simulink model "aavs1_8ap"  (R2013a)
settings: Solver=ode45  StartTime=0.0  StopTime=10.0  RelTol=1e-3
undefined symbols (not defined in the file or in its folder): sfp
libraries: xbsIndex_r4 x1437, casper_library_misc x32, xps_library x17
(part 1 of 11)
settings Model: Creator=jack  LastModifiedBy=jack

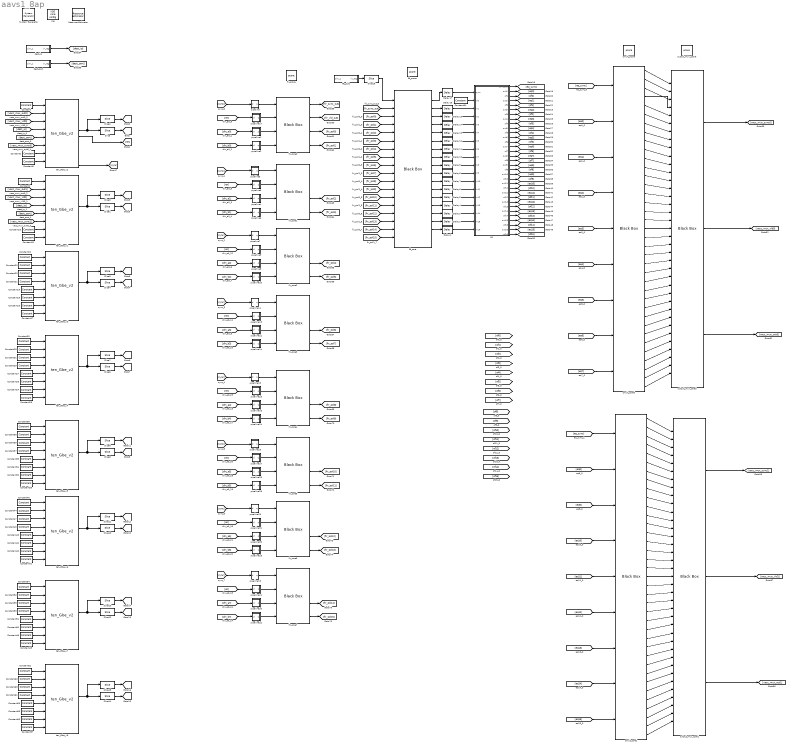
== system aavs1_8ap ==
  " System Generator" : xbsIndex_r4/ System Generator  Tag=genX  xilinxfamily=virtex6  part=xc6vsx475t  speed=-1  package=ff1759  synthesis_tool=XST  clock_wrapper=Clock Enables  directory=./aavs1_8ap/sysgen  proj_type=Project Navigator  Synth_file=XST Defaults  Impl_file=ISE Defaults  testbench=off  simulink_period=1  sysclk_period=5  dcm_input_clock_period=100  incr_netlist=off  trim_vbits=Everywhere in SubSystem  dbl_ovrd=According to Block Masks  core_generation=According to Block Masks  run_coregen=off  deprecated_control=off  eval_field=0  block_type=sysgen
  Constant{,1,18,22..23,26,30..31,34,38..39,42,46..47,50,54..55,58,62..63} (20 alike) : xbsIndex_r4/Constant  const=0  gui_display_data_type=Boolean  arith_type=Boolean  n_bits=16  bin_pt=14  preci_type=Single  exp_width=8  frac_width=24  explicit_period=on  period=1  equ=P=C  opselect=C  inp2=PCIN>>17  opr=+  inp1=P  carry=CIN  dbl_ovrd=off  block_type=constant
  Constant{2..3,10..11,16..17,24..25,32..33,40..41,48..49,56..57,64} (17 alike) : xbsIndex_r4/Constant  const=1  gui_display_data_type=Boolean  arith_type=Boolean  n_bits=16  bin_pt=14  preci_type=Single  exp_width=8  frac_width=24  explicit_period=on  period=1  equ=P=C  opselect=C  inp2=PCIN>>17  opr=+  inp1=P  carry=CIN  dbl_ovrd=off  block_type=constant
  Constant{19,21,27,29,35,37,43,45,51,53,59,61} (12 alike) : xbsIndex_r4/Constant  const=0  gui_display_data_type=Fixed-point  arith_type=Unsigned  n_bits=32  bin_pt=0  preci_type=Single  exp_width=8  frac_width=24  explicit_period=on  period=1  equ=P=C  opselect=C  inp2=PCIN>>17  opr=+  inp1=P  carry=CIN  dbl_ovrd=off  block_type=constant
  Constant{20,28,36,44,52,60} (6 alike) : xbsIndex_r4/Constant  const=0  gui_display_data_type=Fixed-point  arith_type=Unsigned  n_bits=64  bin_pt=0  preci_type=Single  exp_width=8  frac_width=24  explicit_period=on  period=1  equ=P=C  opselect=C  inp2=PCIN>>17  opr=+  inp1=P  carry=CIN  dbl_ovrd=off  block_type=constant
  Delay{1..17} (17 alike) : xbsIndex_r4/Delay  rst=off  infoeditControl=Selection of Reset will increase slice count due to use of real FFs and instead of SRLs  en=off  latency=1  dbl_ovrd=off  reg_retiming=off  block_type=delay
  Resource Estimator : xbsIndex_r4/Resource Estimator  Tag=resEstTag  Slices=0  FFs=0  BRAMs=0  LUTs=0  IOBs=0  EBMs=0  TBUFs=0  xl_use_estimator_area=off  est_options=Estimate  xl_estimator_area=[0 0 0 0 0 0 0]  block_type=resource_estimator
      settings: AttributesFormatString=Resource\nEstimator
  Slice{,1,4,6,8,10,12,14} (8 alike) : xbsIndex_r4/Slice  nbits=32  boolean_output=off  mode=Lower Bit Location + Width  bit1=0  base1=MSB of Input  bit0=0  base0=LSB of Input  dbl_ovrd=off  block_type=slice
  Slice{2..3,5,7,9,11,13,15} (8 alike) : xbsIndex_r4/Slice  nbits=32  boolean_output=off  mode=Lower Bit Location + Width  bit1=0  base1=MSB of Input  bit0=32  base0=LSB of Input  dbl_ovrd=off  block_type=slice
  Slice16 : xbsIndex_r4/Slice  nbits=10  boolean_output=off  mode=Lower Bit Location + Width  bit1=0  base1=MSB of Input  bit0=0  base0=LSB of Input  dbl_ovrd=off  block_type=slice
  cmult_core0 : xbsIndex_r4/Black Box  init_code=cmult_core_config  sim_method=Inactive  verbose=off  block_type=blackbox2
  cmult_core1 : xbsIndex_r4/Black Box  init_code=cmult_core_config  sim_method=Inactive  verbose=off  block_type=blackbox2
  cmult_pcore : xps_library/pcore  Tag=xps:pcore  pcore_path=cmult_core/cmult_core.ngc
  dest_ip : Subsystem  Tag=xps:sw_reg  AncestorBlock=xps_library/software register  mask(swreg){mode=one value, io_dir=From Processor, io_delay=0, sample_period=1, names=reg, bitwidths=32, arith_types=0, bin_pts=0, sim_port=on, show_format=off}
      mask prompts: io_dir "I/O direction"; io_delay "I/O delay"; sample_period "Sample period"; names "Name:"; bitwidths "Bitwidth:"; arith_types "Type (ufix=0, fix=1, bool=2):"; bin_pts "Binary pt:"; sim_port "Provide sim input/output?"; show_format "Print format string?"
      mask init:
      | swreg_init(gcb)
      settings: AttributesFormatString=1input
      mask TypeOptions mode: one value | fields of equal size | fields of arbitrary size
      mask Callback mode: swreg_cb(gcb);
      mask TypeOptions io_dir: To Processor | From Processor
      mask Callback io_dir:
      | mask_enables = get_param(gcb, 'MaskEnables');
      | mask_names = get_param(gcb, 'MaskNames');
      | if strcmp(get_param(gcb, 'io_dir'), 'To Processor'),
      |     mask_enables{ismember(mask_names, 'sample_period')} = 'off';
      | else
      |     mask_enables{ismember(mask_names, 'sample_period')} = 'on';
      | end
      | set_param(gcb, 'MaskEnables', mask_enables);
      mask Callback bitwidths:
      | swreg_maskcheck(gcb);
      | % blk = gcb;
      | % mode = get_param(blk, 'mode');
      | % current_widths = eval(get_param(blk, 'bitwidths'));
      | % if (strcmp(mode, 'one value') || strcmp(mode, 'fields of equal size')) && (length(current_widths) > 1),
      | %     error('Only one width may be specified for this mode.');
      | % elseif strcmp(mode, 'fields of arbitrary size')
      | %     current_names = textscan(strtrim(strrep(strrep(get_param(blk, 'names'), ']', ''), '[', '')), '%s');
      | %     current_names = current_names{1};
      | %     numios = length(current_names);
      | %     if length(current_widths) ~= numios,
      | %         error('%d field names specified, but %d widths?', numios, length(current_widths));
      | %     end
      | % end
      | % total_width = 0;
      | % for ctr = 1 : length(current_widths),
      | %     total_width = total_width + current_widths(ctr);
      | % end
      | % if total_width > 32,
      | %     error('Total width must be 32 or less, set to %d.', total_width);
      | % end
      mask Callback arith_types:
      | [numios, ~, ~, ~, current_types] = swreg_maskcheck(gcb);
      | % blk = gcb;
      | % mode = get_param(blk, 'mode');
      | % current_types = eval(get_param(blk, 'arith_types'));
      | % numios = length(current_types);
      | % if (strcmp(mode, 'one value') || strcmp(mode, 'fields of equal size')) && (length(current_types) > 1),
      | %     error('Only one type may be specified for this mode.');
      | % elseif strcmp(mode, 'fields of arbitrary size')
      | %     current_names = textscan(strtrim(strrep(strrep(get_param(blk, 'names'), ']', ''), '[', '')), '%s');
      | %     current_names = current_names{1};
      | %     numios = length(current_names);
      | %     if length(current_types) ~= numios,
      | %         error('%d field names specified, but %d types?', numios, length(current_types));
      | %     end
      | % end
      | problem = 0;
      | for ctr = 1 : numios,
      |     t = current_types(ctr);
      |     if (t < 0) || (t > 2),
      |         problem = t;
      |         ctr = numios + 1;
      |     end
      | end
      | if problem ~= 0,
      |     error('Type cannot be %i, must be 0, 1 or 2.', problem);
      | end
      mask Callback bin_pts:
      | swreg_maskcheck(gcb);
      | % blk = gcb;
      | % mode = get_param(blk, 'mode');
      | % current_bins = eval(get_param(blk, 'bin_pts'));
      | % if (strcmp(mode, 'one value') || strcmp(mode, 'fields of equal size')) && (length(current_bins) > 1),
      | %     error('Only one binary pt may be specified for this mode.');
      | % elseif strcmp(mode, 'fields of arbitrary size')
      | %     current_names = textscan(strtrim(strrep(strrep(get_param(blk, 'names'), ']', ''), '[', '')), '%s');
      | %     current_names = current_names{1};
      | %     numios = length(current_names);
      | %     if length(current_bins) ~= numios,
      | %         error('%d field names specified, but %d binary pts?', numios, length(current_bins));
      | %     end
      | % end
  dest_port : Subsystem  Tag=xps:sw_reg  AncestorBlock=xps_library/software register  mask(swreg){mode=one value, io_dir=From Processor, io_delay=0, sample_period=1, names=reg, bitwidths=32, arith_types=0, bin_pts=0, sim_port=on, show_format=off}
      mask prompts: io_dir "I/O direction"; io_delay "I/O delay"; sample_period "Sample period"; names "Name:"; bitwidths "Bitwidth:"; arith_types "Type (ufix=0, fix=1, bool=2):"; bin_pts "Binary pt:"; sim_port "Provide sim input/output?"; show_format "Print format string?"
      mask init:
      | swreg_init(gcb)
      settings: AttributesFormatString=1input
      mask TypeOptions mode: one value | fields of equal size | fields of arbitrary size
      mask Callback mode: swreg_cb(gcb);
      mask TypeOptions io_dir: To Processor | From Processor
      mask Callback io_dir:
      | mask_enables = get_param(gcb, 'MaskEnables');
      | mask_names = get_param(gcb, 'MaskNames');
      | if strcmp(get_param(gcb, 'io_dir'), 'To Processor'),
      |     mask_enables{ismember(mask_names, 'sample_period')} = 'off';
      | else
      |     mask_enables{ismember(mask_names, 'sample_period')} = 'on';
      | end
      | set_param(gcb, 'MaskEnables', mask_enables);
      mask Callback bitwidths:
      | swreg_maskcheck(gcb);
      | % blk = gcb;
      | % mode = get_param(blk, 'mode');
      | % current_widths = eval(get_param(blk, 'bitwidths'));
      | % if (strcmp(mode, 'one value') || strcmp(mode, 'fields of equal size')) && (length(current_widths) > 1),
      | %     error('Only one width may be specified for this mode.');
      | % elseif strcmp(mode, 'fields of arbitrary size')
      | %     current_names = textscan(strtrim(strrep(strrep(get_param(blk, 'names'), ']', ''), '[', '')), '%s');
      | %     current_names = current_names{1};
      | %     numios = length(current_names);
      | %     if length(current_widths) ~= numios,
      | %         error('%d field names specified, but %d widths?', numios, length(current_widths));
      | %     end
      | % end
      | % total_width = 0;
      | % for ctr = 1 : length(current_widths),
      | %     total_width = total_width + current_widths(ctr);
      | % end
      | % if total_width > 32,
      | %     error('Total width must be 32 or less, set to %d.', total_width);
      | % end
      mask Callback arith_types:
      | [numios, ~, ~, ~, current_types] = swreg_maskcheck(gcb);
      | % blk = gcb;
      | % mode = get_param(blk, 'mode');
      | % current_types = eval(get_param(blk, 'arith_types'));
      | % numios = length(current_types);
      | % if (strcmp(mode, 'one value') || strcmp(mode, 'fields of equal size')) && (length(current_types) > 1),
      | %     error('Only one type may be specified for this mode.');
      | % elseif strcmp(mode, 'fields of arbitrary size')
      | %     current_names = textscan(strtrim(strrep(strrep(get_param(blk, 'names'), ']', ''), '[', '')), '%s');
      | %     current_names = current_names{1};
      | %     numios = length(current_names);
      | %     if length(current_types) ~= numios,
      | %         error('%d field names specified, but %d types?', numios, length(current_types));
      | %     end
      | % end
      | problem = 0;
      | for ctr = 1 : numios,
      |     t = current_types(ctr);
      |     if (t < 0) || (t > 2),
      |         problem = t;
      |         ctr = numios + 1;
      |     end
      | end
      | if problem ~= 0,
      |     error('Type cannot be %i, must be 0, 1 or 2.', problem);
      | end
      mask Callback bin_pts:
      | swreg_maskcheck(gcb);
      | % blk = gcb;
      | % mode = get_param(blk, 'mode');
      | % current_bins = eval(get_param(blk, 'bin_pts'));
      | % if (strcmp(mode, 'one value') || strcmp(mode, 'fields of equal size')) && (length(current_bins) > 1),
      | %     error('Only one binary pt may be specified for this mode.');
      | % elseif strcmp(mode, 'fields of arbitrary size')
      | %     current_names = textscan(strtrim(strrep(strrep(get_param(blk, 'names'), ']', ''), '[', '')), '%s');
      | %     current_names = current_names{1};
      | %     numios = length(current_names);
      | %     if length(current_bins) ~= numios,
      | %         error('%d field names specified, but %d binary pts?', numios, length(current_bins));
      | %     end
      | % end
  eq : Subsystem
  fft_core : xbsIndex_r4/Black Box  init_code=fft_core_config  sim_method=Inactive  verbose=off  block_type=blackbox2
  fft_pcore : xps_library/pcore  Tag=xps:pcore  pcore_path=fft_core/fft_core.ngc
  fft_shift : Subsystem  Tag=xps:sw_reg  AncestorBlock=xps_library/software register  mask(swreg){mode=one value, io_dir=From Processor, io_delay=0, sample_period=1, names=reg, bitwidths=32, arith_types=0, bin_pts=0, sim_port=on, show_format=off}
      mask prompts: io_dir "I/O direction"; io_delay "I/O delay"; sample_period "Sample period"; names "Name:"; bitwidths "Bitwidth:"; arith_types "Type (ufix=0, fix=1, bool=2):"; bin_pts "Binary pt:"; sim_port "Provide sim input/output?"; show_format "Print format string?"
      mask init:
      | swreg_init(gcb)
      settings: AttributesFormatString=1input
      mask TypeOptions mode: one value | fields of equal size | fields of arbitrary size
      mask Callback mode: swreg_cb(gcb);
      mask TypeOptions io_dir: To Processor | From Processor
      mask Callback io_dir:
      | mask_enables = get_param(gcb, 'MaskEnables');
      | mask_names = get_param(gcb, 'MaskNames');
      | if strcmp(get_param(gcb, 'io_dir'), 'To Processor'),
      |     mask_enables{ismember(mask_names, 'sample_period')} = 'off';
      | else
      |     mask_enables{ismember(mask_names, 'sample_period')} = 'on';
      | end
      | set_param(gcb, 'MaskEnables', mask_enables);
      mask Callback bitwidths:
      | swreg_maskcheck(gcb);
      | % blk = gcb;
      | % mode = get_param(blk, 'mode');
      | % current_widths = eval(get_param(blk, 'bitwidths'));
      | % if (strcmp(mode, 'one value') || strcmp(mode, 'fields of equal size')) && (length(current_widths) > 1),
      | %     error('Only one width may be specified for this mode.');
      | % elseif strcmp(mode, 'fields of arbitrary size')
      | %     current_names = textscan(strtrim(strrep(strrep(get_param(blk, 'names'), ']', ''), '[', '')), '%s');
      | %     current_names = current_names{1};
      | %     numios = length(current_names);
      | %     if length(current_widths) ~= numios,
      | %         error('%d field names specified, but %d widths?', numios, length(current_widths));
      | %     end
      | % end
      | % total_width = 0;
      | % for ctr = 1 : length(current_widths),
      | %     total_width = total_width + current_widths(ctr);
      | % end
      | % if total_width > 32,
      | %     error('Total width must be 32 or less, set to %d.', total_width);
      | % end
      mask Callback arith_types:
      | [numios, ~, ~, ~, current_types] = swreg_maskcheck(gcb);
      | % blk = gcb;
      | % mode = get_param(blk, 'mode');
      | % current_types = eval(get_param(blk, 'arith_types'));
      | % numios = length(current_types);
      | % if (strcmp(mode, 'one value') || strcmp(mode, 'fields of equal size')) && (length(current_types) > 1),
      | %     error('Only one type may be specified for this mode.');
      | % elseif strcmp(mode, 'fields of arbitrary size')
      | %     current_names = textscan(strtrim(strrep(strrep(get_param(blk, 'names'), ']', ''), '[', '')), '%s');
      | %     current_names = current_names{1};
      | %     numios = length(current_names);
      | %     if length(current_types) ~= numios,
      | %         error('%d field names specified, but %d types?', numios, length(current_types));
      | %     end
      | % end
      | problem = 0;
      | for ctr = 1 : numios,
      |     t = current_types(ctr);
      |     if (t < 0) || (t > 2),
      |         problem = t;
      |         ctr = numios + 1;
      |     end
      | end
      | if problem ~= 0,
      |     error('Type cannot be %i, must be 0, 1 or 2.', problem);
      | end
      mask Callback bin_pts:
      | swreg_maskcheck(gcb);
      | % blk = gcb;
      | % mode = get_param(blk, 'mode');
      | % current_bins = eval(get_param(blk, 'bin_pts'));
      | % if (strcmp(mode, 'one value') || strcmp(mode, 'fields of equal size')) && (length(current_bins) > 1),
      | %     error('Only one binary pt may be specified for this mode.');
      | % elseif strcmp(mode, 'fields of arbitrary size')
      | %     current_names = textscan(strtrim(strrep(strrep(get_param(blk, 'names'), ']', ''), '[', '')), '%s');
      | %     current_names = current_names{1};
      | %     numios = length(current_names);
      | %     if length(current_bins) ~= numios,
      | %         error('%d field names specified, but %d binary pts?', numios, length(current_bins));
      | %     end
      | % end
  fir_core{0..7} (8 alike) : xbsIndex_r4/Black Box  init_code=fir_core_config  sim_method=Inactive  verbose=off  block_type=blackbox2
  fir_pcore : xps_library/pcore  Tag=xps:pcore  pcore_path=fir_core/fir_core.ngc
  output_mux_core0 : xbsIndex_r4/Black Box  init_code=output_mux_core_config  sim_method=Inactive  verbose=off  block_type=blackbox2
  output_mux_core1 : xbsIndex_r4/Black Box  init_code=output_mux_core_config  sim_method=Inactive  verbose=off  block_type=blackbox2
  output_mux_pcore : xps_library/pcore  Tag=xps:pcore  pcore_path=output_mux_core/output_mux_core.ngc
  pipeline : Subsystem  AncestorBlock=casper_library_delays/pipeline  mask(pipeline){latency=1}
      mask help:
      | An explicitly laid-out delay line to avoid mapping to SRL16s
      | for use in pipelining to help achieve timing closure.
      mask init:
      | pipeline_init(gcb,'latency',latency);
      settings: AttributesFormatString=Latency = %<latency>
      mask Display:
      | port_label('input', 1, 'd');
      | port_label('output', 1, 'q');
      | disp(['Z^-', num2str(latency)]);
  pipeline1 : Subsystem  AncestorBlock=casper_library_delays/pipeline  mask(pipeline){latency=1}
      mask help:
      | An explicitly laid-out delay line to avoid mapping to SRL16s
      | for use in pipelining to help achieve timing closure.
      mask init:
      | pipeline_init(gcb,'latency',latency);
      settings: AttributesFormatString=Latency = %<latency>
      mask Display:
      | port_label('input', 1, 'd');
      | port_label('output', 1, 'q');
      | disp(['Z^-', num2str(latency)]);
  pipeline10 : Subsystem  AncestorBlock=casper_library_delays/pipeline  mask(pipeline){latency=1}
      mask help:
      | An explicitly laid-out delay line to avoid mapping to SRL16s
      | for use in pipelining to help achieve timing closure.
      mask init:
      | pipeline_init(gcb,'latency',latency);
      settings: AttributesFormatString=Latency = %<latency>
      mask Display:
      | port_label('input', 1, 'd');
      | port_label('output', 1, 'q');
      | disp(['Z^-', num2str(latency)]);
  pipeline11 : Subsystem  AncestorBlock=casper_library_delays/pipeline  mask(pipeline){latency=1}
      mask help:
      | An explicitly laid-out delay line to avoid mapping to SRL16s
      | for use in pipelining to help achieve timing closure.
      mask init:
      | pipeline_init(gcb,'latency',latency);
      settings: AttributesFormatString=Latency = %<latency>
      mask Display:
      | port_label('input', 1, 'd');
      | port_label('output', 1, 'q');
      | disp(['Z^-', num2str(latency)]);
  pipeline12 : Subsystem  AncestorBlock=casper_library_delays/pipeline  mask(pipeline){latency=1}
      mask help:
      | An explicitly laid-out delay line to avoid mapping to SRL16s
      | for use in pipelining to help achieve timing closure.
      mask init:
      | pipeline_init(gcb,'latency',latency);
      settings: AttributesFormatString=Latency = %<latency>
      mask Display:
      | port_label('input', 1, 'd');
      | port_label('output', 1, 'q');
      | disp(['Z^-', num2str(latency)]);
  pipeline13 : Subsystem  AncestorBlock=casper_library_delays/pipeline  mask(pipeline){latency=1}
      mask help:
      | An explicitly laid-out delay line to avoid mapping to SRL16s
      | for use in pipelining to help achieve timing closure.
      mask init:
      | pipeline_init(gcb,'latency',latency);
      settings: AttributesFormatString=Latency = %<latency>
      mask Display:
      | port_label('input', 1, 'd');
      | port_label('output', 1, 'q');
      | disp(['Z^-', num2str(latency)]);
  pipeline14 : Subsystem  AncestorBlock=casper_library_delays/pipeline  mask(pipeline){latency=1}
      mask help:
      | An explicitly laid-out delay line to avoid mapping to SRL16s
      | for use in pipelining to help achieve timing closure.
      mask init:
      | pipeline_init(gcb,'latency',latency);
      settings: AttributesFormatString=Latency = %<latency>
      mask Display:
      | port_label('input', 1, 'd');
      | port_label('output', 1, 'q');
      | disp(['Z^-', num2str(latency)]);
  pipeline15 : Subsystem  AncestorBlock=casper_library_delays/pipeline  mask(pipeline){latency=1}
      mask help:
      | An explicitly laid-out delay line to avoid mapping to SRL16s
      | for use in pipelining to help achieve timing closure.
      mask init:
      | pipeline_init(gcb,'latency',latency);
      settings: AttributesFormatString=Latency = %<latency>
      mask Display:
      | port_label('input', 1, 'd');
      | port_label('output', 1, 'q');
      | disp(['Z^-', num2str(latency)]);
  pipeline16 : Subsystem  AncestorBlock=casper_library_delays/pipeline  mask(pipeline){latency=1}
      mask help:
      | An explicitly laid-out delay line to avoid mapping to SRL16s
      | for use in pipelining to help achieve timing closure.
      mask init:
      | pipeline_init(gcb,'latency',latency);
      settings: AttributesFormatString=Latency = %<latency>
      mask Display:
      | port_label('input', 1, 'd');
      | port_label('output', 1, 'q');
      | disp(['Z^-', num2str(latency)]);
  pipeline17 : Subsystem  AncestorBlock=casper_library_delays/pipeline  mask(pipeline){latency=1}
      mask help:
      | An explicitly laid-out delay line to avoid mapping to SRL16s
      | for use in pipelining to help achieve timing closure.
      mask init:
      | pipeline_init(gcb,'latency',latency);
      settings: AttributesFormatString=Latency = %<latency>
      mask Display:
      | port_label('input', 1, 'd');
      | port_label('output', 1, 'q');
      | disp(['Z^-', num2str(latency)]);
  pipeline18 : Subsystem  AncestorBlock=casper_library_delays/pipeline  mask(pipeline){latency=1}
      mask help:
      | An explicitly laid-out delay line to avoid mapping to SRL16s
      | for use in pipelining to help achieve timing closure.
      mask init:
      | pipeline_init(gcb,'latency',latency);
      settings: AttributesFormatString=Latency = %<latency>
      mask Display:
      | port_label('input', 1, 'd');
      | port_label('output', 1, 'q');
      | disp(['Z^-', num2str(latency)]);
  pipeline19 : Subsystem  AncestorBlock=casper_library_delays/pipeline  mask(pipeline){latency=1}
      mask help:
      | An explicitly laid-out delay line to avoid mapping to SRL16s
      | for use in pipelining to help achieve timing closure.
      mask init:
      | pipeline_init(gcb,'latency',latency);
      settings: AttributesFormatString=Latency = %<latency>
      mask Display:
      | port_label('input', 1, 'd');
      | port_label('output', 1, 'q');
      | disp(['Z^-', num2str(latency)]);
  pipeline2 : Subsystem  AncestorBlock=casper_library_delays/pipeline  mask(pipeline){latency=1}
      mask help:
      | An explicitly laid-out delay line to avoid mapping to SRL16s
      | for use in pipelining to help achieve timing closure.
      mask init:
      | pipeline_init(gcb,'latency',latency);
      settings: AttributesFormatString=Latency = %<latency>
      mask Display:
      | port_label('input', 1, 'd');
      | port_label('output', 1, 'q');
      | disp(['Z^-', num2str(latency)]);
  pipeline20 : Subsystem  AncestorBlock=casper_library_delays/pipeline  mask(pipeline){latency=1}
      mask help:
      | An explicitly laid-out delay line to avoid mapping to SRL16s
      | for use in pipelining to help achieve timing closure.
      mask init:
      | pipeline_init(gcb,'latency',latency);
      settings: AttributesFormatString=Latency = %<latency>
      mask Display:
      | port_label('input', 1, 'd');
      | port_label('output', 1, 'q');
      | disp(['Z^-', num2str(latency)]);
  pipeline21 : Subsystem  AncestorBlock=casper_library_delays/pipeline  mask(pipeline){latency=1}
      mask help:
      | An explicitly laid-out delay line to avoid mapping to SRL16s
      | for use in pipelining to help achieve timing closure.
      mask init:
      | pipeline_init(gcb,'latency',latency);
      settings: AttributesFormatString=Latency = %<latency>
      mask Display:
      | port_label('input', 1, 'd');
      | port_label('output', 1, 'q');
      | disp(['Z^-', num2str(latency)]);
  pipeline22 : Subsystem  AncestorBlock=casper_library_delays/pipeline  mask(pipeline){latency=1}
      mask help:
      | An explicitly laid-out delay line to avoid mapping to SRL16s
      | for use in pipelining to help achieve timing closure.
      mask init:
      | pipeline_init(gcb,'latency',latency);
      settings: AttributesFormatString=Latency = %<latency>
      mask Display:
      | port_label('input', 1, 'd');
      | port_label('output', 1, 'q');
      | disp(['Z^-', num2str(latency)]);
  pipeline23 : Subsystem  AncestorBlock=casper_library_delays/pipeline  mask(pipeline){latency=1}
      mask help:
      | An explicitly laid-out delay line to avoid mapping to SRL16s
      | for use in pipelining to help achieve timing closure.
      mask init:
      | pipeline_init(gcb,'latency',latency);
      settings: AttributesFormatString=Latency = %<latency>
      mask Display:
      | port_label('input', 1, 'd');
      | port_label('output', 1, 'q');
      | disp(['Z^-', num2str(latency)]);
  pipeline24 : Subsystem  AncestorBlock=casper_library_delays/pipeline  mask(pipeline){latency=1}
      mask help:
      | An explicitly laid-out delay line to avoid mapping to SRL16s
      | for use in pipelining to help achieve timing closure.
      mask init:
      | pipeline_init(gcb,'latency',latency);
      settings: AttributesFormatString=Latency = %<latency>
      mask Display:
      | port_label('input', 1, 'd');
      | port_label('output', 1, 'q');
      | disp(['Z^-', num2str(latency)]);
  pipeline25 : Subsystem  AncestorBlock=casper_library_delays/pipeline  mask(pipeline){latency=1}
      mask help:
      | An explicitly laid-out delay line to avoid mapping to SRL16s
      | for use in pipelining to help achieve timing closure.
      mask init:
      | pipeline_init(gcb,'latency',latency);
      settings: AttributesFormatString=Latency = %<latency>
      mask Display:
      | port_label('input', 1, 'd');
      | port_label('output', 1, 'q');
      | disp(['Z^-', num2str(latency)]);
  pipeline26 : Subsystem  AncestorBlock=casper_library_delays/pipeline  mask(pipeline){latency=1}
      mask help:
      | An explicitly laid-out delay line to avoid mapping to SRL16s
      | for use in pipelining to help achieve timing closure.
      mask init:
      | pipeline_init(gcb,'latency',latency);
      settings: AttributesFormatString=Latency = %<latency>
      mask Display:
      | port_label('input', 1, 'd');
      | port_label('output', 1, 'q');
      | disp(['Z^-', num2str(latency)]);
  pipeline27 : Subsystem  AncestorBlock=casper_library_delays/pipeline  mask(pipeline){latency=1}
      mask help:
      | An explicitly laid-out delay line to avoid mapping to SRL16s
      | for use in pipelining to help achieve timing closure.
      mask init:
      | pipeline_init(gcb,'latency',latency);
      settings: AttributesFormatString=Latency = %<latency>
      mask Display:
      | port_label('input', 1, 'd');
      | port_label('output', 1, 'q');
      | disp(['Z^-', num2str(latency)]);
  pipeline28 : Subsystem  AncestorBlock=casper_library_delays/pipeline  mask(pipeline){latency=1}
      mask help:
      | An explicitly laid-out delay line to avoid mapping to SRL16s
      | for use in pipelining to help achieve timing closure.
      mask init:
      | pipeline_init(gcb,'latency',latency);
      settings: AttributesFormatString=Latency = %<latency>
      mask Display:
      | port_label('input', 1, 'd');
      | port_label('output', 1, 'q');
      | disp(['Z^-', num2str(latency)]);
  pipeline29 : Subsystem  AncestorBlock=casper_library_delays/pipeline  mask(pipeline){latency=1}
      mask help:
      | An explicitly laid-out delay line to avoid mapping to SRL16s
      | for use in pipelining to help achieve timing closure.
      mask init:
      | pipeline_init(gcb,'latency',latency);
      settings: AttributesFormatString=Latency = %<latency>
      mask Display:
      | port_label('input', 1, 'd');
      | port_label('output', 1, 'q');
      | disp(['Z^-', num2str(latency)]);
  pipeline3 : Subsystem  AncestorBlock=casper_library_delays/pipeline  mask(pipeline){latency=1}
      mask help:
      | An explicitly laid-out delay line to avoid mapping to SRL16s
      | for use in pipelining to help achieve timing closure.
      mask init:
      | pipeline_init(gcb,'latency',latency);
      settings: AttributesFormatString=Latency = %<latency>
      mask Display:
      | port_label('input', 1, 'd');
      | port_label('output', 1, 'q');
      | disp(['Z^-', num2str(latency)]);
  pipeline30 : Subsystem  AncestorBlock=casper_library_delays/pipeline  mask(pipeline){latency=1}
      mask help:
      | An explicitly laid-out delay line to avoid mapping to SRL16s
      | for use in pipelining to help achieve timing closure.
      mask init:
      | pipeline_init(gcb,'latency',latency);
      settings: AttributesFormatString=Latency = %<latency>
      mask Display:
      | port_label('input', 1, 'd');
      | port_label('output', 1, 'q');
      | disp(['Z^-', num2str(latency)]);
  pipeline31 : Subsystem  AncestorBlock=casper_library_delays/pipeline  mask(pipeline){latency=1}
      mask help:
      | An explicitly laid-out delay line to avoid mapping to SRL16s
      | for use in pipelining to help achieve timing closure.
      mask init:
      | pipeline_init(gcb,'latency',latency);
      settings: AttributesFormatString=Latency = %<latency>
      mask Display:
      | port_label('input', 1, 'd');
      | port_label('output', 1, 'q');
      | disp(['Z^-', num2str(latency)]);
  pipeline4 : Subsystem  AncestorBlock=casper_library_delays/pipeline  mask(pipeline){latency=1}
      mask help:
      | An explicitly laid-out delay line to avoid mapping to SRL16s
      | for use in pipelining to help achieve timing closure.
      mask init:
      | pipeline_init(gcb,'latency',latency);
      settings: AttributesFormatString=Latency = %<latency>
      mask Display:
      | port_label('input', 1, 'd');
      | port_label('output', 1, 'q');
      | disp(['Z^-', num2str(latency)]);
  pipeline5 : Subsystem  AncestorBlock=casper_library_delays/pipeline  mask(pipeline){latency=1}
      mask help:
      | An explicitly laid-out delay line to avoid mapping to SRL16s
      | for use in pipelining to help achieve timing closure.
      mask init:
      | pipeline_init(gcb,'latency',latency);
      settings: AttributesFormatString=Latency = %<latency>
      mask Display:
      | port_label('input', 1, 'd');
      | port_label('output', 1, 'q');
      | disp(['Z^-', num2str(latency)]);
  pipeline6 : Subsystem  AncestorBlock=casper_library_delays/pipeline  mask(pipeline){latency=1}
      mask help:
      | An explicitly laid-out delay line to avoid mapping to SRL16s
      | for use in pipelining to help achieve timing closure.
      mask init:
      | pipeline_init(gcb,'latency',latency);
      settings: AttributesFormatString=Latency = %<latency>
      mask Display:
      | port_label('input', 1, 'd');
      | port_label('output', 1, 'q');
      | disp(['Z^-', num2str(latency)]);
  pipeline7 : Subsystem  AncestorBlock=casper_library_delays/pipeline  mask(pipeline){latency=1}
      mask help:
      | An explicitly laid-out delay line to avoid mapping to SRL16s
      | for use in pipelining to help achieve timing closure.
      mask init:
      | pipeline_init(gcb,'latency',latency);
      settings: AttributesFormatString=Latency = %<latency>
      mask Display:
      | port_label('input', 1, 'd');
      | port_label('output', 1, 'q');
      | disp(['Z^-', num2str(latency)]);
  pipeline8 : Subsystem  AncestorBlock=casper_library_delays/pipeline  mask(pipeline){latency=1}
      mask help:
      | An explicitly laid-out delay line to avoid mapping to SRL16s
      | for use in pipelining to help achieve timing closure.
      mask init:
      | pipeline_init(gcb,'latency',latency);
      settings: AttributesFormatString=Latency = %<latency>
      mask Display:
      | port_label('input', 1, 'd');
      | port_label('output', 1, 'q');
      | disp(['Z^-', num2str(latency)]);
  pipeline9 : Subsystem  AncestorBlock=casper_library_delays/pipeline  mask(pipeline){latency=1}
      mask help:
      | An explicitly laid-out delay line to avoid mapping to SRL16s
      | for use in pipelining to help achieve timing closure.
      mask init:
      | pipeline_init(gcb,'latency',latency);
      settings: AttributesFormatString=Latency = %<latency>
      mask Display:
      | port_label('input', 1, 'd');
      | port_label('output', 1, 'q');
      | disp(['Z^-', num2str(latency)]);
  ten_Gbe_v1 : xps_library/ten_Gbe_v2  Tag=xps:tengbe_v2  flavour=sfp+  slot=0  port_r1=0  port_r2_cx4=0  port_r2_sfpp=1  rx_dist_ram=on  large_frames=off  show_param=off  pre_emph_r2=1.07  pre_emph=3  post_emph_r2=0.18  rxeqmix_r2=7  swing_r2=940  swing=800  fab_en=on  fab_mac=hex2dec('123456780000')  fab_ip=192*(2^24) + 168*(2^16) + 5*(2^8) + 20*(2^0)  fab_udp=10000  fab_gate=1  cpu_rx_en=on  cpu_tx_en=on  ttl=hex2dec('FF')  promisc_mode=off  txctr=off  txerrctr=off  txerrctr_len=100  txofctr=off  txfullctr=off  txvldctr=off  txsnaplen=0 - no snap  rxctr=off  rxerrctr=off  rxerrctr_len=100  rxofctr=off  rxbadctr=off  rxvldctr=off  rxeofctr=off  rxsnaplen=0 - no snap
  ten_Gbe_v2 : xps_library/ten_Gbe_v2  Tag=xps:tengbe_v2  flavour=sfp+  slot=0  port_r1=0  port_r2_cx4=0  port_r2_sfpp=0  rx_dist_ram=on  large_frames=off  show_param=off  pre_emph_r2=1.07  pre_emph=3  post_emph_r2=0.18  rxeqmix_r2=7  swing_r2=940  swing=800  fab_en=on  fab_mac=hex2dec('123456780000')  fab_ip=192*(2^24) + 168*(2^16) + 5*(2^8) + 20*(2^0)  fab_udp=10000  fab_gate=1  cpu_rx_en=on  cpu_tx_en=on  ttl=hex2dec('FF')  promisc_mode=off  txctr=off  txerrctr=off  txerrctr_len=100  txofctr=off  txfullctr=off  txvldctr=off  txsnaplen=0 - no snap  rxctr=off  rxerrctr=off  rxerrctr_len=100  rxofctr=off  rxbadctr=off  rxvldctr=off  rxeofctr=off  rxsnaplen=0 - no snap
  ten_Gbe_v3 : xps_library/ten_Gbe_v2  Tag=xps:tengbe_v2  flavour=sfp+  slot=0  port_r1=0  port_r2_cx4=0  port_r2_sfpp=2  rx_dist_ram=on  large_frames=off  show_param=off  pre_emph_r2=1.07  pre_emph=3  post_emph_r2=0.18  rxeqmix_r2=7  swing_r2=940  swing=800  fab_en=on  fab_mac=hex2dec('123456780000')  fab_ip=192*(2^24) + 168*(2^16) + 5*(2^8) + 20*(2^0)  fab_udp=10000  fab_gate=1  cpu_rx_en=on  cpu_tx_en=on  ttl=hex2dec('FF')  promisc_mode=off  txctr=off  txerrctr=off  txerrctr_len=100  txofctr=off  txfullctr=off  txvldctr=off  txsnaplen=0 - no snap  rxctr=off  rxerrctr=off  rxerrctr_len=100  rxofctr=off  rxbadctr=off  rxvldctr=off  rxeofctr=off  rxsnaplen=0 - no snap
  ten_Gbe_v4 : xps_library/ten_Gbe_v2  Tag=xps:tengbe_v2  flavour=sfp+  slot=0  port_r1=0  port_r2_cx4=0  port_r2_sfpp=3  rx_dist_ram=on  large_frames=off  show_param=off  pre_emph_r2=1.07  pre_emph=3  post_emph_r2=0.18  rxeqmix_r2=7  swing_r2=940  swing=800  fab_en=on  fab_mac=hex2dec('123456780000')  fab_ip=192*(2^24) + 168*(2^16) + 5*(2^8) + 20*(2^0)  fab_udp=10000  fab_gate=1  cpu_rx_en=on  cpu_tx_en=on  ttl=hex2dec('FF')  promisc_mode=off  txctr=off  txerrctr=off  txerrctr_len=100  txofctr=off  txfullctr=off  txvldctr=off  txsnaplen=0 - no snap  rxctr=off  rxerrctr=off  rxerrctr_len=100  rxofctr=off  rxbadctr=off  rxvldctr=off  rxeofctr=off  rxsnaplen=0 - no snap
  ten_Gbe_v5 : xps_library/ten_Gbe_v2  Tag=xps:tengbe_v2  flavour=sfp+  slot=1  port_r1=0  port_r2_cx4=0  port_r2_sfpp=0  rx_dist_ram=on  large_frames=off  show_param=off  pre_emph_r2=1.07  pre_emph=3  post_emph_r2=0.18  rxeqmix_r2=7  swing_r2=940  swing=800  fab_en=on  fab_mac=hex2dec('123456780000')  fab_ip=192*(2^24) + 168*(2^16) + 5*(2^8) + 20*(2^0)  fab_udp=10000  fab_gate=1  cpu_rx_en=on  cpu_tx_en=on  ttl=hex2dec('FF')  promisc_mode=off  txctr=off  txerrctr=off  txerrctr_len=100  txofctr=off  txfullctr=off  txvldctr=off  txsnaplen=0 - no snap  rxctr=off  rxerrctr=off  rxerrctr_len=100  rxofctr=off  rxbadctr=off  rxvldctr=off  rxeofctr=off  rxsnaplen=0 - no snap
  ten_Gbe_v6 : xps_library/ten_Gbe_v2  Tag=xps:tengbe_v2  flavour=sfp+  slot=1  port_r1=0  port_r2_cx4=0  port_r2_sfpp=1  rx_dist_ram=on  large_frames=off  show_param=off  pre_emph_r2=1.07  pre_emph=3  post_emph_r2=0.18  rxeqmix_r2=7  swing_r2=940  swing=800  fab_en=on  fab_mac=hex2dec('123456780000')  fab_ip=192*(2^24) + 168*(2^16) + 5*(2^8) + 20*(2^0)  fab_udp=10000  fab_gate=1  cpu_rx_en=on  cpu_tx_en=on  ttl=hex2dec('FF')  promisc_mode=off  txctr=off  txerrctr=off  txerrctr_len=100  txofctr=off  txfullctr=off  txvldctr=off  txsnaplen=0 - no snap  rxctr=off  rxerrctr=off  rxerrctr_len=100  rxofctr=off  rxbadctr=off  rxvldctr=off  rxeofctr=off  rxsnaplen=0 - no snap
  ten_Gbe_v7 : xps_library/ten_Gbe_v2  Tag=xps:tengbe_v2  flavour=sfp+  slot=1  port_r1=0  port_r2_cx4=0  port_r2_sfpp=2  rx_dist_ram=on  large_frames=off  show_param=off  pre_emph_r2=1.07  pre_emph=3  post_emph_r2=0.18  rxeqmix_r2=7  swing_r2=940  swing=800  fab_en=on  fab_mac=hex2dec('123456780000')  fab_ip=192*(2^24) + 168*(2^16) + 5*(2^8) + 20*(2^0)  fab_udp=10000  fab_gate=1  cpu_rx_en=on  cpu_tx_en=on  ttl=hex2dec('FF')  promisc_mode=off  txctr=off  txerrctr=off  txerrctr_len=100  txofctr=off  txfullctr=off  txvldctr=off  txsnaplen=0 - no snap  rxctr=off  rxerrctr=off  rxerrctr_len=100  rxofctr=off  rxbadctr=off  rxvldctr=off  rxeofctr=off  rxsnaplen=0 - no snap
  ten_Gbe_v8 : xps_library/ten_Gbe_v2  Tag=xps:tengbe_v2  flavour=sfp+  slot=1  port_r1=0  port_r2_cx4=0  port_r2_sfpp=3  rx_dist_ram=on  large_frames=off  show_param=off  pre_emph_r2=1.07  pre_emph=3  post_emph_r2=0.18  rxeqmix_r2=7  swing_r2=940  swing=800  fab_en=on  fab_mac=hex2dec('123456780000')  fab_ip=192*(2^24) + 168*(2^16) + 5*(2^8) + 20*(2^0)  fab_udp=10000  fab_gate=1  cpu_rx_en=on  cpu_tx_en=on  ttl=hex2dec('FF')  promisc_mode=off  txctr=off  txerrctr=off  txerrctr_len=100  txofctr=off  txfullctr=off  txvldctr=off  txsnaplen=0 - no snap  rxctr=off  rxerrctr=off  rxerrctr_len=100  rxofctr=off  rxbadctr=off  rxvldctr=off  rxeofctr=off  rxsnaplen=0 - no snap
  xsg : xps_library/XSG core config  Tag=xps:xsg  hw_sys=ROACH2:sx475t  clk_src=sys_clk  ROACH_clk_src=sys_clk  ROACH2_clk_src=sys_clk  MKDIG_clk_src=sys_clk  clk_rate=200  sample_period=1  synthesis_tool=XST
  wires:
  ten_Gbe_v2/6 -> Slice2/1, Slice/1
  Slice/1 -> [din_a0]
  Slice2/1 -> [din_b0]
  [sync] -> pipeline/1(d)
  ten_Gbe_v2/7 -> [en]
  [en] -> pipeline17/1(d)
  ten_Gbe_v1/6 -> Slice1/1, Slice3/1
  Slice1/1 -> [din_a1]
  Slice3/1 -> [din_b1]
  ten_Gbe_v3/6 -> Slice5/1, Slice4/1
  Slice4/1 -> [din_a2]
  Slice5/1 -> [din_b2]
  ten_Gbe_v4/6 -> Slice7/1, Slice6/1
  Slice6/1 -> [din_a3]
  Slice7/1 -> [din_b3]
  ten_Gbe_v5/6 -> Slice9/1, Slice8/1
  Slice8/1 -> [din_a4]
  Slice9/1 -> [din_b4]
  ten_Gbe_v6/6 -> Slice10/1, Slice11/1
  Slice10/1 -> [din_a5]
  Slice11/1 -> [din_b5]
  ten_Gbe_v7/6 -> Slice12/1, Slice13/1
  Slice12/1 -> [din_a6]
  Slice13/1 -> [din_b6]
  ten_Gbe_v8/6 -> Slice14/1, Slice15/1
  Slice14/1 -> [din_a7]
  Slice15/1 -> [din_b7]
  fft_core/1 -> Delay17/1
  Constant/1 -> ten_Gbe_v2/1
  Constant2/1 -> ten_Gbe_v2/7
  Constant3/1 -> ten_Gbe_v2/8
  [vacc_mux_sync0] -> ten_Gbe_v2/6
  [dest_port] -> ten_Gbe_v2/5
  [dest_ip] -> ten_Gbe_v2/4
  Constant1/1 -> ten_Gbe_v1/1
  [vacc_mux_vld1] -> ten_Gbe_v1/3
  Constant10/1 -> ten_Gbe_v1/7
  Constant11/1 -> ten_Gbe_v1/8
  [vacc_mux_sync1] -> ten_Gbe_v1/6
  [dest_port] -> ten_Gbe_v1/5
  [vacc_mux_out1] -> ten_Gbe_v1/2
  [dest_ip] -> ten_Gbe_v1/4
  Constant22/1 -> ten_Gbe_v3/1
  Constant23/1 -> ten_Gbe_v3/3
  Constant16/1 -> ten_Gbe_v3/7
  Constant17/1 -> ten_Gbe_v3/8
  Constant18/1 -> ten_Gbe_v3/6
  Constant19/1 -> ten_Gbe_v3/5
  Constant20/1 -> ten_Gbe_v3/2
  Constant21/1 -> ten_Gbe_v3/4
  Constant30/1 -> ten_Gbe_v4/1
  Constant31/1 -> ten_Gbe_v4/3
  Constant24/1 -> ten_Gbe_v4/7
  Constant25/1 -> ten_Gbe_v4/8
  Constant26/1 -> ten_Gbe_v4/6
  Constant27/1 -> ten_Gbe_v4/5
  Constant28/1 -> ten_Gbe_v4/2
  Constant29/1 -> ten_Gbe_v4/4
  Constant38/1 -> ten_Gbe_v5/1
  Constant39/1 -> ten_Gbe_v5/3
  Constant32/1 -> ten_Gbe_v5/7
  Constant33/1 -> ten_Gbe_v5/8
  Constant34/1 -> ten_Gbe_v5/6
  Constant35/1 -> ten_Gbe_v5/5
  Constant36/1 -> ten_Gbe_v5/2
  Constant37/1 -> ten_Gbe_v5/4
  Constant46/1 -> ten_Gbe_v6/1
  Constant47/1 -> ten_Gbe_v6/3
  Constant40/1 -> ten_Gbe_v6/7
  Constant41/1 -> ten_Gbe_v6/8
  Constant42/1 -> ten_Gbe_v6/6
  Constant43/1 -> ten_Gbe_v6/5
  Constant44/1 -> ten_Gbe_v6/2
  Constant45/1 -> ten_Gbe_v6/4
  Constant54/1 -> ten_Gbe_v7/1
  Constant55/1 -> ten_Gbe_v7/3
  Constant48/1 -> ten_Gbe_v7/7
  Constant49/1 -> ten_Gbe_v7/8
  Constant50/1 -> ten_Gbe_v7/6
  Constant51/1 -> ten_Gbe_v7/5
  Constant52/1 -> ten_Gbe_v7/2
  Constant53/1 -> ten_Gbe_v7/4
  Constant62/1 -> ten_Gbe_v8/1
  Constant63/1 -> ten_Gbe_v8/3
  Constant56/1 -> ten_Gbe_v8/7
  Constant57/1 -> ten_Gbe_v8/8
  Constant58/1 -> ten_Gbe_v8/6
  Constant59/1 -> ten_Gbe_v8/5
  Constant60/1 -> ten_Gbe_v8/2
  Constant61/1 -> ten_Gbe_v8/4
  ten_Gbe_v2/12 -> [sync]
  pipeline/1(q) -> fir_core0/1
  pipeline17/1(q) -> fir_core0/2
  Constant64/1 -> eq/2(vld)
  fft_core/7 -> Delay11/1
  fft_core/2 -> Delay16/1
  fft_core/3 -> Delay15/1
  fft_core/4 -> Delay14/1
  fft_core/5 -> Delay13/1
  fft_core/6 -> Delay12/1
  fft_core/8 -> Delay10/1
  fft_core/9 -> Delay9/1
  fft_core/10 -> Delay8/1
  fft_core/11 -> Delay7/1
  fft_core/12 -> Delay6/1
  fft_core/13 -> Delay5/1
  fft_core/14 -> Delay4/1
  fft_core/15 -> Delay3/1
  fft_core/16 -> Delay2/1
  fft_core/17 -> Delay1/1
  eq/1(sync_out) -> [eq_sync]
  eq/31(of15) -> [of14]
  eq/22(out11) -> [eq10]
  eq/13(of6) -> [of5]
  eq/23(of11) -> [of10]
  eq/21(of10) -> [of9]
  eq/15(of7) -> [of6]
  eq/16(out8) -> [eq7]
  eq/6(out3) -> [eq2]
  eq/29(of14) -> [of13]
  eq/8(out4) -> [eq3]
  eq/5(of2) -> [of1]
  eq/28(out14) -> [eq13]
  eq/11(of5) -> [of4]
  eq/30(out15) -> [eq14]
  eq/27(of13) -> [of12]
  eq/14(out7) -> [eq6]
  eq/32(out16) -> [eq15]
  eq/19(of9) -> [of8]
  eq/26(out13) -> [eq12]
  eq/4(out2) -> [eq1]
  eq/20(out10) -> [eq9]
  eq/9(of4) -> [of3]
  eq/33(of16) -> [of15]
  eq/18(out9) -> [eq8]
  eq/12(out6) -> [eq5]
  eq/25(of12) -> [of11]
  eq/7(of3) -> [of2]
  eq/10(out5) -> [eq4]
  eq/24(out12) -> [eq11]
  eq/2(out1) -> [eq0]
  eq/3(of1) -> [of0]
  eq/17(of8) -> [of7]
  [eq_sync] -> cmult_core0/1
  [eq0] -> cmult_core0/2
  [eq4] -> cmult_core0/6
  [eq3] -> cmult_core0/5
  [eq6] -> cmult_core0/8
  [eq5] -> cmult_core0/7
  [eq7] -> cmult_core0/9
  [eq2] -> cmult_core0/4
  [eq1] -> cmult_core0/3
  [eq12] -> cmult_core1/6
  [eq10] -> cmult_core1/4
  [eq14] -> cmult_core1/8
  [eq8] -> cmult_core1/2
  [eq13] -> cmult_core1/7
  [eq11] -> cmult_core1/5
  [eq9] -> cmult_core1/3
  [eq_sync] -> cmult_core1/1
  [eq15] -> cmult_core1/9
  output_mux_core0/3 -> [vacc_mux_out0]
  output_mux_core0/2 -> [vacc_mux_vld0]
  output_mux_core0/1 -> [vacc_mux_sync0]
  dest_ip/1(in_reg) -> [dest_ip]
  dest_port/1(in_reg) -> [dest_port]
  [din_a0] -> pipeline1/1(d)
  pipeline1/1(q) -> fir_core0/3
  [din_b0] -> pipeline2/1(d)
  pipeline2/1(q) -> fir_core0/4
  [sync] -> pipeline3/1(d)
  [en] -> pipeline5/1(d)
  pipeline3/1(q) -> fir_core1/1
  pipeline5/1(q) -> fir_core1/2
  [din_a1] -> pipeline4/1(d)
  pipeline4/1(q) -> fir_core1/3
  [din_b1] -> pipeline6/1(d)
  pipeline6/1(q) -> fir_core1/4
  [sync] -> pipeline7/1(d)
  [en] -> pipeline9/1(d)
  pipeline7/1(q) -> fir_core2/1
  pipeline9/1(q) -> fir_core2/2
  [din_a2] -> pipeline8/1(d)
  pipeline8/1(q) -> fir_core2/3
  [din_b2] -> pipeline10/1(d)
  pipeline10/1(q) -> fir_core2/4
  [sync] -> pipeline11/1(d)
  [en] -> pipeline13/1(d)
  pipeline11/1(q) -> fir_core3/1
  pipeline13/1(q) -> fir_core3/2
  [din_a3] -> pipeline12/1(d)
  pipeline12/1(q) -> fir_core3/3
  [din_b3] -> pipeline14/1(d)
  pipeline14/1(q) -> fir_core3/4
  [sync] -> pipeline15/1(d)
  [en] -> pipeline23/1(d)
  pipeline15/1(q) -> fir_core4/1
  pipeline23/1(q) -> fir_core4/2
  [din_a4] -> pipeline16/1(d)
  pipeline16/1(q) -> fir_core4/3
  [din_b4] -> pipeline24/1(d)
  pipeline24/1(q) -> fir_core4/4
  [sync] -> pipeline25/1(d)
  [en] -> pipeline27/1(d)
  pipeline25/1(q) -> fir_core5/1
  pipeline27/1(q) -> fir_core5/2
  [din_a5] -> pipeline26/1(d)
  pipeline26/1(q) -> fir_core5/3
  [din_b5] -> pipeline28/1(d)
  pipeline28/1(q) -> fir_core5/4
  [sync] -> pipeline29/1(d)
  [en] -> pipeline31/1(d)
  pipeline29/1(q) -> fir_core6/1
  pipeline31/1(q) -> fir_core6/2
  [din_a6] -> pipeline30/1(d)
  pipeline30/1(q) -> fir_core6/3
  [din_b6] -> pipeline18/1(d)
  pipeline18/1(q) -> fir_core6/4
  [sync] -> pipeline19/1(d)
  [en] -> pipeline21/1(d)
  pipeline19/1(q) -> fir_core7/1
  pipeline21/1(q) -> fir_core7/2
  [din_a7] -> pipeline20/1(d)
  pipeline20/1(q) -> fir_core7/3
  [din_b7] -> pipeline22/1(d)
  pipeline22/1(q) -> fir_core7/4
  fir_core0/1 -> [fir_sync_out]
  fir_core0/2 -> [fir_vld_out]
  fir_core0/3 -> [fir_pol0]
  fir_core0/4 -> [fir_pol1]
  fir_core1/3 -> [fir_pol2]
  fir_core1/4 -> [fir_pol3]
  fir_core2/3 -> [fir_pol4]
  fir_core2/4 -> [fir_pol5]
  fir_core3/3 -> [fir_pol6]
  fir_core3/4 -> [fir_pol7]
  fir_core4/3 -> [fir_pol8]
  fir_core4/4 -> [fir_pol9]
  fir_core5/3 -> [fir_pol10]
  fir_core5/4 -> [fir_pol11]
  fir_core6/3 -> [fir_pol12]
  fir_core6/4 -> [fir_pol13]
  fir_core7/3 -> [fir_pol14]
  fir_core7/4 -> [fir_pol15]
  fft_shift/1(in_reg) -> Slice16/1
  [fir_pol4] -> fft_core/7
  [fir_pol11] -> fft_core/14
  [fir_pol10] -> fft_core/13
  [fir_pol7] -> fft_core/10
  [fir_pol9] -> fft_core/12
  [fir_pol13] -> fft_core/16
  [fir_pol3] -> fft_core/6
  [fir_sync_out] -> fft_core/2
  [fir_pol6] -> fft_core/9
  [fir_pol0] -> fft_core/3
  [fir_pol12] -> fft_core/15
  [fir_pol5] -> fft_core/8
  [fir_pol14] -> fft_core/17
  [fir_pol15] -> fft_core/18
  [fir_pol1] -> fft_core/4
  [fir_pol8] -> fft_core/11
  [fir_pol2] -> fft_core/5
  cmult_core0/4 -> output_mux_core0/4
  cmult_core0/3 -> output_mux_core0/3
  cmult_core0/5 -> output_mux_core0/5
  cmult_core0/2 -> output_mux_core0/2
  cmult_core0/6 -> output_mux_core0/6
  cmult_core0/1 -> output_mux_core0/1
  cmult_core0/7 -> output_mux_core0/7
  cmult_core0/8 -> output_mux_core0/8
  cmult_core0/9 -> output_mux_core0/9
  cmult_core0/10 -> output_mux_core0/10
  cmult_core0/11 -> output_mux_core0/11
  cmult_core0/12 -> output_mux_core0/12
  cmult_core0/13 -> output_mux_core0/13
  cmult_core0/14 -> output_mux_core0/14
  cmult_core0/15 -> output_mux_core0/15
  cmult_core0/16 -> output_mux_core0/16
  cmult_core0/17 -> output_mux_core0/17
  cmult_core0/18 -> output_mux_core0/18
  cmult_core0/19 -> output_mux_core0/19
  cmult_core0/20 -> output_mux_core0/20
  cmult_core0/21 -> output_mux_core0/21
  cmult_core0/22 -> output_mux_core0/22
  cmult_core0/23 -> output_mux_core0/23
  cmult_core0/24 -> output_mux_core0/24
  cmult_core0/25 -> output_mux_core0/25
  cmult_core0/26 -> output_mux_core0/26
  cmult_core0/27 -> output_mux_core0/27
  cmult_core0/28 -> output_mux_core0/28
  cmult_core0/29 -> output_mux_core0/29
  cmult_core0/30 -> output_mux_core0/30
  cmult_core0/31 -> output_mux_core0/31
  cmult_core0/32 -> output_mux_core0/32
  cmult_core0/33 -> output_mux_core0/33
  cmult_core0/37 -> output_mux_core0/37
  cmult_core0/36 -> output_mux_core0/36
  cmult_core0/34 -> output_mux_core0/34
  cmult_core0/35 -> output_mux_core0/35
  cmult_core1/37 -> output_mux_core1/37
  cmult_core1/26 -> output_mux_core1/26
  cmult_core1/6 -> output_mux_core1/6
  cmult_core1/35 -> output_mux_core1/35
  cmult_core1/36 -> output_mux_core1/36
  cmult_core1/22 -> output_mux_core1/22
  cmult_core1/34 -> output_mux_core1/34
  cmult_core1/15 -> output_mux_core1/15
  cmult_core1/21 -> output_mux_core1/21
  cmult_core1/19 -> output_mux_core1/19
  cmult_core1/4 -> output_mux_core1/4
  cmult_core1/5 -> output_mux_core1/5
  cmult_core1/12 -> output_mux_core1/12
  cmult_core1/14 -> output_mux_core1/14
  cmult_core1/30 -> output_mux_core1/30
  cmult_core1/31 -> output_mux_core1/31
  cmult_core1/13 -> output_mux_core1/13
  cmult_core1/25 -> output_mux_core1/25
  cmult_core1/27 -> output_mux_core1/27
  cmult_core1/8 -> output_mux_core1/8
  cmult_core1/17 -> output_mux_core1/17
  cmult_core1/20 -> output_mux_core1/20
  cmult_core1/10 -> output_mux_core1/10
  cmult_core1/9 -> output_mux_core1/9
  cmult_core1/1 -> output_mux_core1/1
  cmult_core1/29 -> output_mux_core1/29
  cmult_core1/28 -> output_mux_core1/28
  cmult_core1/32 -> output_mux_core1/32
  cmult_core1/24 -> output_mux_core1/24
  cmult_core1/7 -> output_mux_core1/7
  cmult_core1/2 -> output_mux_core1/2
  cmult_core1/11 -> output_mux_core1/11
  cmult_core1/33 -> output_mux_core1/33
  cmult_core1/3 -> output_mux_core1/3
  cmult_core1/16 -> output_mux_core1/16
  cmult_core1/23 -> output_mux_core1/23
  cmult_core1/18 -> output_mux_core1/18
  output_mux_core1/1 -> [vacc_mux_sync1]
  output_mux_core1/2 -> [vacc_mux_vld1]
  output_mux_core1/3 -> [vacc_mux_out1]
  Slice16/1 -> fft_core/1
  [vacc_mux_out0] -> ten_Gbe_v2/2
  [vacc_mux_vld0] -> ten_Gbe_v2/3
  Delay1/1 -> eq/18(in16)
  Delay2/1 -> eq/17(in15)
  Delay3/1 -> eq/16(in14)
  Delay4/1 -> eq/15(in13)
  Delay5/1 -> eq/14(in12)
  Delay6/1 -> eq/13(in11)
  Delay7/1 -> eq/12(in10)
  Delay8/1 -> eq/11(in9)
  Delay9/1 -> eq/10(in8)
  Delay10/1 -> eq/9(in7)
  Delay11/1 -> eq/8(in6)
  Delay12/1 -> eq/7(in5)
  Delay13/1 -> eq/6(in4)
  Delay14/1 -> eq/5(in3)
  Delay15/1 -> eq/4(in2)
  Delay16/1 -> eq/3(in1)
  Delay17/1 -> eq/1(sync)
